simulink model "nakamura_1"  (R2021b)
settings: Solver=VariableStepAuto  StartTime=0.0  StopTime=30  RelTol=1e-3
values from neighbouring files (symbols this model uses):
  c = inv(N) * (xT-x0)    [nakamura.m]
  u1 = (x1T - x10)/T    (= 0.2)    [nakamura.m]
  x10 = 1    [nakamura.m]
  x20 = 2    [nakamura.m]
  x30 = 3    [nakamura.m]
settings Model: Creator=mbober  LastModifiedBy=mbober

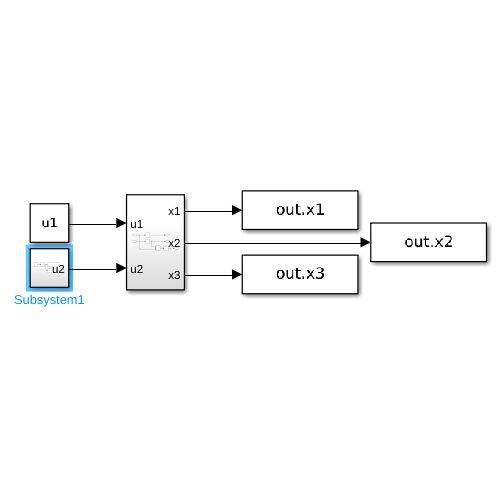
[thumbnail: Simulink's stored preview of the top-level diagram]
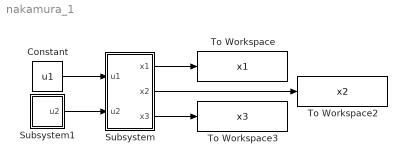
== system nakamura_1 ==
  Constant : Constant  Value=u1
  Subsystem : Subsystem
  Subsystem1 : Subsystem
  To Workspace : ToWorkspace  VariableName=x1  SampleTime=-1
  To Workspace2 : ToWorkspace  VariableName=x2  SampleTime=-1
  To Workspace3 : ToWorkspace  VariableName=x3  SampleTime=-1
  wires:
  Subsystem1/1(u2) -> Subsystem/2(u2)
  Subsystem/1(x1) -> To Workspace/1
  Subsystem/2(x2) -> To Workspace2/1
  Subsystem/3(x3) -> To Workspace3/1
  Constant/1 -> Subsystem/1(u1)

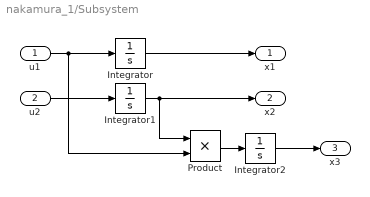
== system nakamura_1/Subsystem ==
  u1 : Inport
  u2 : Inport  Port=2
  Integrator : Integrator  InitialCondition=x10
  Integrator1 : Integrator  InitialCondition=x20
  Integrator2 : Integrator  InitialCondition=x30
  Product : Product
  x1 : Outport
  x2 : Outport  Port=2
  x3 : Outport  Port=3
  wires:
  Integrator2/1 -> x3/1
  u1/1 -> Product/2, Integrator/1
  Integrator1/1 -> Product/1, x2/1
  Product/1 -> Integrator2/1
  Integrator/1 -> x1/1
  u2/1 -> Integrator1/1

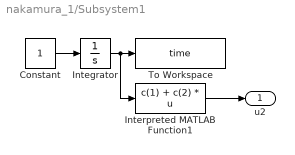
== system nakamura_1/Subsystem1 ==
  Constant : Constant
  Integrator : Integrator
  Interpreted MATLAB Function1 : MATLABFcn  MATLABFcn=c(1) + c(2) * u
  To Workspace : ToWorkspace  VariableName=time  SampleTime=-1
  u2 : Outport
  wires:
  Interpreted MATLAB Function1/1 -> u2/1
  Constant/1 -> Integrator/1
  Integrator/1 -> Interpreted MATLAB Function1/1, To Workspace/1
